simulink model "simu"  (R2016a)
settings: Solver=VariableStepAuto  StartTime=0.0  StopTime=10.0  RelTol=1e-3
settings Model: Creator=Fulvio  LastModifiedBy=Fulvio
settings SFSimCC: SimCustomSourceCode=|
  | file.c
  | gnu.c
  | mathLib.c
  | vigaLib.c
  | vigaForzado.c
  | vigaEDO.c
  | viga.c
settings SFSimCC: SimCustomHeaderCode=|
  | #include "file.h"
  | #include "gnu.h"
  | #include 'mathLib.h"
  | #include "vigaLib.h"
  | #include "vigaForzado.h"
  | #include "vigaEDO.h"
  | #include "viga.h"h"

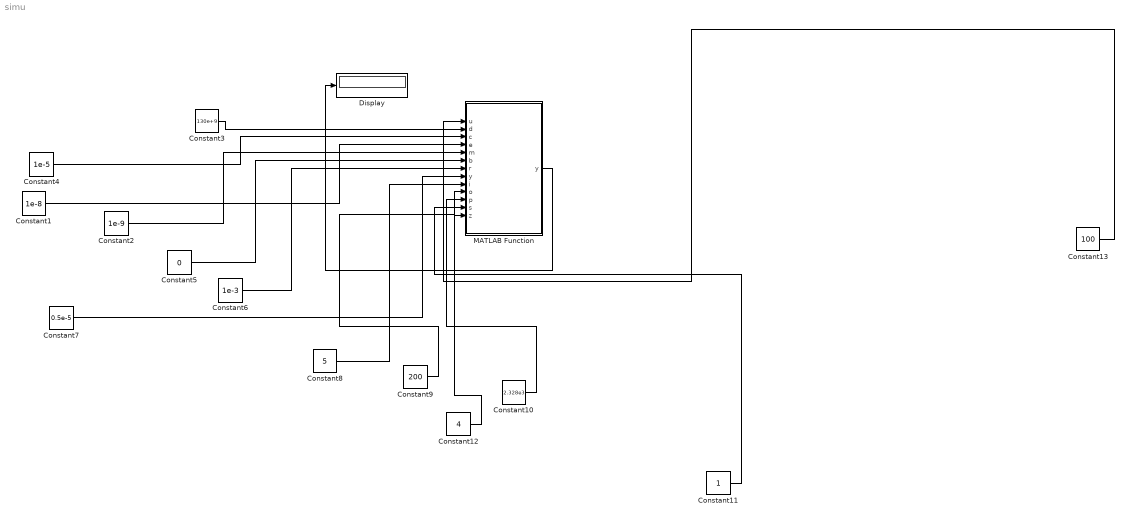
== system simu ==
  Constant1 : Constant  Value=1e-8
  Constant10 : Constant  Value=2.328e3
  Constant11 : Constant
  Constant12 : Constant  Value=4
  Constant13 : Constant  Value=100
  Constant2 : Constant  Value=1e-9
  Constant3 : Constant  Value=130e+9
  Constant4 : Constant  Value=1e-5
  Constant5 : Constant  Value=0
  Constant6 : Constant  Value=1e-3
  Constant7 : Constant  Value=0.5e-5
  Constant8 : Constant  Value=5
  Constant9 : Constant  Value=200
  Display : Display
  MATLAB Function : MATLAB Function  TreatAsAtomicUnit=on
  wires:
  Constant13/1 -> MATLAB Function/1(u)
  MATLAB Function/1(y) -> Display/1
  Constant2/1 -> MATLAB Function/5(m)
  Constant1/1 -> MATLAB Function/4(e)
  Constant3/1 -> MATLAB Function/2(d)
  Constant4/1 -> MATLAB Function/3(c)
  Constant5/1 -> MATLAB Function/6(b)
  Constant6/1 -> MATLAB Function/7(r)
  Constant7/1 -> MATLAB Function/8("y ")
  Constant8/1 -> MATLAB Function/9(i)
  Constant9/1 -> MATLAB Function/10(o)
  Constant10/1 -> MATLAB Function/11(p)
  Constant11/1 -> MATLAB Function/12(s)
  Constant12/1 -> MATLAB Function/13(z)

== matlab function simu/MATLAB Function ==
  data: u input; y output; d input; c input; e input; m input; b input; r input; y input; i input; o input; p input; s input; z input
function y = fcn(u,d,c,e,m,b,r,y,i,o,p,s,z)
%#codegen
y = 0.0;
y = coder.ceval('viga',u,d,c,e,m);
